simulink model "Save"  (R2020b)
settings: Solver=VariableStepAuto  StartTime=0.0  StopTime=10.0  RelTol=1e-3
values from neighbouring files (symbols this model uses):
  A_2 = [0  0  0; 0  0  0; 0  0  0]    [Angular_gust.mat]    (also in Linear_gust.mat; Real_Values.m = zeros(3); Trial_Script.m = zeros(3); TryingNewAeroCoeffs.m = zeros(3))
  A_AD = [0 0 0 0 0 0 0 0 0 0 0 0 ... (36 elements, 6x6)]    [Angular_gust.mat]    (also in Linear_gust.mat; Real_Values.m = horzcat(A_i, A_ii); Trial_Script.m = horzcat(A_i, A_ii); TryingNewAeroCoeffs.m = horzcat(A_i, A_ii))
  A_kal = [0 0 0 0 0 0 0 0 0 0 0 0 ... (36 elements, 6x6)]    [Angular_gust.mat]    (also in Linear_gust.mat; Real_Values.m = [0 0 0 1 0 0; Trial_Script.m = [0 0 0 1 0 0; TryingNewAeroCoeffs.m = [0 0 0 1 0 0)
  B_2 = [0.0024294842205  2.57653534931e-06  6.44659625064e-05; 0  -0.000916808772026  -2.10833406567e-07; 0  0  -0.000799328564006]    [Angular_gust.mat]    (also in Linear_gust.mat; Real_Values.m = I_inv; Trial_Script.m = I_inv; TryingNewAeroCoeffs.m = I_inv)
  B_AD = [0 0 0 0 0 0 0 0 0 0 0 0 ... (36 elements, 6x6)]    [Angular_gust.mat]    (also in Linear_gust.mat; Real_Values.m = horzcat(B_i, B_ii); Trial_Script.m = horzcat(B_i, B_ii); TryingNewAeroCoeffs.m = horzcat(B_i, B_ii))
  B_kal = [0 0 0 0 0 0 0 0 0 0 0 0 ... (36 elements, 6x6)]    [Angular_gust.mat]    (also in Linear_gust.mat; Real_Values.m = [0 0 0 0 0 0; Trial_Script.m = [0 0 0 0 0 0; TryingNewAeroCoeffs.m = [0 0 0 0 0 0)
  C_2 = [1  0  0; 0  1  0; 0  0  1]    [Angular_gust.mat]    (also in Linear_gust.mat; Real_Values.m = eye(3); Trial_Script.m = eye(3); TryingNewAeroCoeffs.m = eye(3))
  C_AD = [1 0 0 0 0 0 0 1 0 0 0 0 ... (36 elements, 6x6)]    [Angular_gust.mat]    (also in Linear_gust.mat; Real_Values.m = eye(6); Trial_Script.m = eye(6); TryingNewAeroCoeffs.m = eye(6))
  C_D = 0.6    [Angular_gust.mat]    (also in Linear_gust.mat; Real_Values.m; Trial_Script.m; TryingNewAeroCoeffs.m)
  C_kal = [1 0 0 0 0 0 0 1 0 0 0 0 ... (36 elements, 6x6)]    [Angular_gust.mat]    (also in Linear_gust.mat; Real_Values.m = eye(6); Trial_Script.m = eye(6); TryingNewAeroCoeffs.m = eye(6))
  D_2 = [0  0  0; 0  0  0; 0  0  0]    [Angular_gust.mat]    (also in Linear_gust.mat; Real_Values.m = zeros(3); Trial_Script.m = zeros(3); TryingNewAeroCoeffs.m = zeros(3))
  D_AD = [0 0 0 0 0 0 0 0 0 0 0 0 ... (36 elements, 6x6)]    [Angular_gust.mat]    (also in Linear_gust.mat; Real_Values.m = zeros(6); Trial_Script.m = zeros(6); TryingNewAeroCoeffs.m = zeros(6))
  D_kal = [0 0 0 0 0 0 0 0 0 0 0 0 ... (36 elements, 6x6)]    [Angular_gust.mat]    (also in Linear_gust.mat; Real_Values.m = zeros(6); Trial_Script.m = zeros(6); TryingNewAeroCoeffs.m = zeros(6))
  delta_time = 0.0178961433409    [Angular_gust.mat]    (also in Linear_gust.mat; Real_Values.m = time/length(xdata); Trial_Script.m = time/length(xdata); TryingNewAeroCoeffs.m = time/length(xdata))
  Fb1_l = -2600    [Angular_gust.mat]    (also in Linear_gust.mat; Real_Values.m = -260; Trial_Script.m; TryingNewAeroCoeffs.m)
  Fb1_u = 2600    [Angular_gust.mat]    (also in Linear_gust.mat; Real_Values.m = 260; Trial_Script.m; TryingNewAeroCoeffs.m)
  Fb2_l = -2600    [Angular_gust.mat]    (also in Linear_gust.mat; Real_Values.m = -260; Trial_Script.m; TryingNewAeroCoeffs.m)
  Fb2_u = 2600    [Angular_gust.mat]    (also in Linear_gust.mat; Real_Values.m = 260; Trial_Script.m; TryingNewAeroCoeffs.m)
  Fb3_l = -3200    [Angular_gust.mat]    (also in Linear_gust.mat; Real_Values.m = -320; Trial_Script.m; TryingNewAeroCoeffs.m)
  Fb3_u = 3200    [Angular_gust.mat]    (also in Linear_gust.mat; Real_Values.m = 320; Trial_Script.m; TryingNewAeroCoeffs.m)
  Fb4_l = -3200    [Angular_gust.mat]    (also in Linear_gust.mat; Real_Values.m = -320; Trial_Script.m; TryingNewAeroCoeffs.m)
  Fb4_u = 3200    [Angular_gust.mat]    (also in Linear_gust.mat; Real_Values.m = 320; Trial_Script.m; TryingNewAeroCoeffs.m)
  Fc1_l = -300    [Angular_gust.mat]    (also in Linear_gust.mat; Real_Values.m = -100; Trial_Script.m = -3000; TryingNewAeroCoeffs.m)
  Fc1_u = 300    [Angular_gust.mat]    (also in Linear_gust.mat; Real_Values.m = 100; Trial_Script.m = 3000; TryingNewAeroCoeffs.m)
  Fc2_l = -300    [Angular_gust.mat]    (also in Linear_gust.mat; Real_Values.m = -100; Trial_Script.m = -3000; TryingNewAeroCoeffs.m)
  Fc2_u = 300    [Angular_gust.mat]    (also in Linear_gust.mat; Real_Values.m = 100; Trial_Script.m = 3000; TryingNewAeroCoeffs.m)
  Fc3_l = -300    [Angular_gust.mat]    (also in Linear_gust.mat; Real_Values.m = -100; Trial_Script.m = -3000; TryingNewAeroCoeffs.m)
  Fc3_u = 300    [Angular_gust.mat]    (also in Linear_gust.mat; Real_Values.m = 100; Trial_Script.m = 3000; TryingNewAeroCoeffs.m)
  Ft1_l = -5600    [Angular_gust.mat]    (also in Linear_gust.mat; Real_Values.m = -560; Trial_Script.m; TryingNewAeroCoeffs.m)
  Ft1_u = 5600    [Angular_gust.mat]    (also in Linear_gust.mat; Real_Values.m = 560; Trial_Script.m; TryingNewAeroCoeffs.m)
  Ft2_l = -5600    [Angular_gust.mat]    (also in Linear_gust.mat; Real_Values.m = -560; Trial_Script.m; TryingNewAeroCoeffs.m)
  Ft2_u = 5600    [Angular_gust.mat]    (also in Linear_gust.mat; Real_Values.m = 560; Trial_Script.m; TryingNewAeroCoeffs.m)
  Ft3_l = -3200    [Angular_gust.mat]    (also in Linear_gust.mat; Real_Values.m = -320; Trial_Script.m; TryingNewAeroCoeffs.m)
  Ft3_u = 3200    [Angular_gust.mat]    (also in Linear_gust.mat; Real_Values.m = 320; Trial_Script.m; TryingNewAeroCoeffs.m)
  Ft4_l = -3200    [Angular_gust.mat]    (also in Linear_gust.mat; Real_Values.m = -320; Trial_Script.m; TryingNewAeroCoeffs.m)
  Ft4_u = 3200    [Angular_gust.mat]    (also in Linear_gust.mat; Real_Values.m = 320; Trial_Script.m; TryingNewAeroCoeffs.m)
  g = 9.81    [Angular_gust.mat]    (also in Linear_gust.mat; Real_Values.m; Trial_Script.m; TryingNewAeroCoeffs.m)
  m = 941.102    [Angular_gust.mat]    (also in Linear_gust.mat; Real_Values.m; Trial_Script.m = 645; TryingNewAeroCoeffs.m)
  r_0 = [0 0 0]    [Angular_gust.mat]    (also in Linear_gust.mat; Real_Values.m = [0;0;0]; Trial_Script.m = [0;0;0]; TryingNewAeroCoeffs.m = [0;0;0])
  r_cgCatia = [0.0401998 0.00180957 -0.293434]    [Angular_gust.mat]    (also in Linear_gust.mat; Real_Values.m = TcgCatia*r_cgCatia; Trial_Script.m = [2; 0; 0]; TryingNewAeroCoeffs.m = TcgCatia*r_cgCatia)
  rho = 1.225    [Angular_gust.mat]    (also in Linear_gust.mat; Real_Values.m; Trial_Script.m; TryingNewAeroCoeffs.m)
  S = 1.8    [Angular_gust.mat]    (also in Linear_gust.mat; Real_Values.m; Trial_Script.m; TryingNewAeroCoeffs.m)
  t_finalgust = 17.9140394843    [Angular_gust.mat]    (also in Linear_gust.mat; Real_Values.m = time; TryingNewAeroCoeffs.m = time)
  TcgCatia = [1  0  0; 0  -1  0; 0  0  -1]    [Angular_gust.mat]    (also in Linear_gust.mat; Real_Values.m = [1 0 0; Trial_Script.m = [1 0 0; TryingNewAeroCoeffs.m = [1 0 0)
  theta_0 = [0 0 0]    [Angular_gust.mat]    (also in Linear_gust.mat; Real_Values.m = [0;0;0]; Trial_Script.m = [0;0;0]; TryingNewAeroCoeffs.m = [0;0;0])
  time_delay = 0.01    [Angular_gust.mat]    (also in Linear_gust.mat; Real_Values.m = 0.1; Trial_Script.m = 0.1; TryingNewAeroCoeffs.m)
  Tzy_Shard = [6.12323399574e-17  1  1.22464679915e-16; 1  -6.12323399574e-17  -7.49879891331e-33; 0  1.22464679915e-16  -1]    [Angular_gust.mat]    (also in Linear_gust.mat; Real_Values.m = [cos(pi/2) -sin(pi/2) 0; sin(pi/2) cos(pi/2) 0; 0 0 1]*[1 0 ; Trial_Script.m = [cos(pi/2) -sin(pi/2) 0; sin(pi/2) cos(pi/2) 0; 0 0 1]*[1 0 ; TryingNewAeroCoeffs.m = [cos(pi/2) -sin(pi/2) 0; sin(pi/2) cos(pi/2) 0; 0 0 1]*[1 0 )
  u0_final = 23.9559    [Angular_gust.mat]    (also in Linear_gust.mat; Real_Values.m = u_0(length(u_0)); TryingNewAeroCoeffs.m = u_0(length(u_0)))
  u1_final = -0.480858    [Angular_gust.mat]    (also in Linear_gust.mat; Real_Values.m = u_1(length(u_1)); TryingNewAeroCoeffs.m = u_1(length(u_1)))
  u2_final = -0.725589    [Angular_gust.mat]    (also in Linear_gust.mat; Real_Values.m = u_2(length(u_2)); TryingNewAeroCoeffs.m = u_2(length(u_2)))
  u_0 = [24.7775 24.7775 24.7775 24.7775 24.7775 24.7775 24.7775 24.7775 24.7775 24.7775 24.7775 24.7775 ... (1001 elements, 1001x1)]    [Angular_gust.mat]    (also in Linear_gust.mat; Real_Values.m = a(1:d_shard,1); Trial_Script.m = a(1:d_shard,1); TryingNewAeroCoeffs.m = a(1:d_shard,1))
  u_1 = [0.712897 0.712897 0.712897 0.712897 0.712897 0.712897 0.712897 0.712897 0.712897 0.712897 0.712897 0.712897 ... (1001 elements, 1001x1)]    [Angular_gust.mat]    (also in Linear_gust.mat; Real_Values.m = a(1:d_shard,2); Trial_Script.m = a(1:d_shard,2); TryingNewAeroCoeffs.m = a(1:d_shard,2))
  u_2 = [-0.504815 -0.504815 -0.504815 -0.504815 -0.504815 -0.504815 -0.504815 -0.504815 -0.504815 -0.504815 -0.504815 -0.504815 ... (1001 elements, 1001x1)]    [Angular_gust.mat]    (also in Linear_gust.mat; Real_Values.m = a(1:d_shard,3); Trial_Script.m = a(1:d_shard,3); TryingNewAeroCoeffs.m = a(1:d_shard,3))
  v_0 = [0 0 0]    [Angular_gust.mat]    (also in Linear_gust.mat; Real_Values.m = [0;0;0]; Trial_Script.m = [0;0;0]; TryingNewAeroCoeffs.m = [0;0;0])
  ZI_Cx = [4.10002314469 4.10486511138 4.10970707807 4.11454904475 4.11939101144 4.12423297813 4.12907494481 4.1339169115 4.13875887819 4.14360084487 4.14844281156 4.15328477825 ... (65341 elements, 361x181)]    [Angular_gust.mat]    (also in Linear_gust.mat; Real_Values.m = model_Cx(XI_Cx, YI_Cx); Trial_Script.m = model_Cx(XI_Cx, YI_Cx); TryingNewAeroCoeffs.m = model_Cx(XI_Cx, YI_Cx))
  ZI_Cy = [5.10662222372 5.15407485934 5.20152749496 5.24898013059 5.29643276621 5.34388540184 5.39133803746 5.43879067308 5.48624330871 5.53369594433 5.58114857996 5.62860121558 ... (65341 elements, 361x181)]    [Angular_gust.mat]    (also in Linear_gust.mat; Real_Values.m = model_Cy(XI_Cy, YI_Cy); Trial_Script.m = model_Cy(XI_Cy, YI_Cy); TryingNewAeroCoeffs.m = model_Cy(XI_Cy, YI_Cy))
  ZI_Cz = [-10.5947720774 -10.6317912004 -10.6688103235 -10.7058294465 -10.7428485695 -10.7798676926 -10.8168868156 -10.8539059387 -10.8909250617 -10.9279441847 -10.9649633078 -11.0019824308 ... (65341 elements, 361x181)]    [Angular_gust.mat]    (also in Linear_gust.mat; Real_Values.m = model_Cz(XI_Cz, YI_Cz); Trial_Script.m = model_Cz(XI_Cz, YI_Cz); TryingNewAeroCoeffs.m = model_Cz(XI_Cz, YI_Cz))
  ZI_p = [6.05111971338 6.06712776392 6.08313581446 6.099143865 6.11515191553 6.13115996607 6.14716801661 6.16317606715 6.17918411769 6.19519216823 6.21120021877 6.22720826931 ... (65341 elements, 361x181)]    [Angular_gust.mat]    (also in Linear_gust.mat; Real_Values.m = model_p(XI_p, YI_p); Trial_Script.m = model_p(XI_p, YI_p); TryingNewAeroCoeffs.m = model_p(XI_p, YI_p))
  ZI_q = [0.071083987219 0.054175962948 0.0372679386771 0.0203599144061 0.00345189013513 -0.0134561341358 -0.0303641584068 -0.0472721826778 -0.0641802069487 -0.0810882312197 -0.0979962554907 -0.114904279762 ... (65341 elements, 361x181)]    [Angular_gust.mat]    (also in Linear_gust.mat; Real_Values.m = model_q(XI_q, YI_q); Trial_Script.m = model_q(XI_q, YI_q); TryingNewAeroCoeffs.m = model_q(XI_q, YI_q))
  ZI_r = [-1.8762921931 -1.88364224017 -1.89099228723 -1.8983423343 -1.90569238136 -1.91304242842 -1.92039247549 -1.92774252255 -1.93509256961 -1.94244261668 -1.94979266374 -1.95714271081 ... (65341 elements, 361x181)]    [Angular_gust.mat]    (also in Linear_gust.mat; Real_Values.m = model_r(XI_r, YI_r); Trial_Script.m = model_r(XI_r, YI_r); TryingNewAeroCoeffs.m = model_r(XI_r, YI_r))
undefined symbols (not defined in the file or in its folder): Continuous, Time
libraries: dspsigops x11, simulink x7, pid_lib x3, fuzblock x3, dspindex x3, ctrlSharedLib x2, sharedutil x1, mpclib x1, dspmathops x1, cstblocks x1
(part 2 of 2)

== system Save/Propulsion commands module/Subsystem4 ==
  In1 : Inport
  Fy_actual : Inport  Port=2
  Fz_actual : Inport  Port=3
  In4 : Inport  Port=4
  In5 : Inport  Port=5
  In6 : Inport  Port=6
  T_Vd : Inport  Port=7
  Constant : Constant  Value=[0;1;1]
  Matrix Multiply : Product  Multiplication=Matrix(*)
  Mux : Mux  Inputs=3
  Mux1 : Mux  Inputs=3
  Product : Product
  Scope : Scope
  F_c : Outport
  y : Outport  Port=2
  wires:
  In1/1 -> Mux/1
  Fy_actual/1 -> Mux/2
  Fz_actual/1 -> Mux/3
  Product/1 -> Scope/1, F_c/1  "Fc(t-tau)_actual"
  Mux/1 -> Matrix Multiply/2
  Mux1/1 -> y/1  "Mc(t-tau)_actual"
  In4/1 -> Mux1/1  "M_x_acc"
  In5/1 -> Mux1/2  "M_y_acc"
  In6/1 -> Mux1/3  "M_z_acc"
  T_Vd/1 -> Matrix Multiply/1
  Constant/1 -> Product/1
  Matrix Multiply/1 -> Product/2  "Fc(t-tau)_actual"

== system Save/Propulsion commands module/Top and Bottom including weight counteraction ==
  F_b : Inport
  In2 : Inport  Port=2
  Add : Sum
  Add1 : Sum
  Constant : Constant  Value=m*g
  Gain : Gain  Gain=1/8
  Mux : Mux
  Scope : Scope
  To Workspace : ToWorkspace  VariableName=Ft_inclift  SaveFormat=Timeseries  SampleTime=-1
  To Workspace1 : ToWorkspace  VariableName=Fb_inclift  SaveFormat=Timeseries  SampleTime=-1
  wires:
  Constant/1 -> Mux/4, Mux/3, Mux/2, Mux/1
  Add1/1 -> To Workspace1/1
  F_b/1 -> Add1/1  "F_b"
  In2/1 -> Add/1  "F_t"
  Add/1 -> Scope/1, To Workspace/1
  Gain/1 -> Add1/2, Add/2
  Mux/1 -> Gain/1

== system Save/Subsystem/Drag1 ==
  note: Change to C_D and S per side
  In1 : Inport
  Constant1 : Constant  Value=2
  Constant4 : Constant  Value=0.5*rho*C_D*S
  Demux : Demux  Outputs=3
  Gain : Gain  Gain=0
  Mux : Mux  Inputs=3
  Power : Math  Operator=pow  SaturateOnIntegerOverflow=on
  Power1 : Math  Operator=pow  SaturateOnIntegerOverflow=on
  Power2 : Math  Operator=pow  SaturateOnIntegerOverflow=on
  Product1 : Product
  Out1 : Outport
  drag : Outport  Port=2
  wires:
  Constant1/1 -> Power2/2, Power1/2, Power/2
  Power2/1 -> Mux/3
  Power/1 -> Gain/1
  In1/1 -> Demux/1
  Demux/1 -> Power/1
  Demux/3 -> Power2/1
  Demux/2 -> Power1/1
  Power1/1 -> Mux/2
  Constant4/1 -> Product1/2
  Mux/1 -> Out1/1, Product1/1
  Product1/1 -> drag/1  "drag"
  Gain/1 -> Mux/1

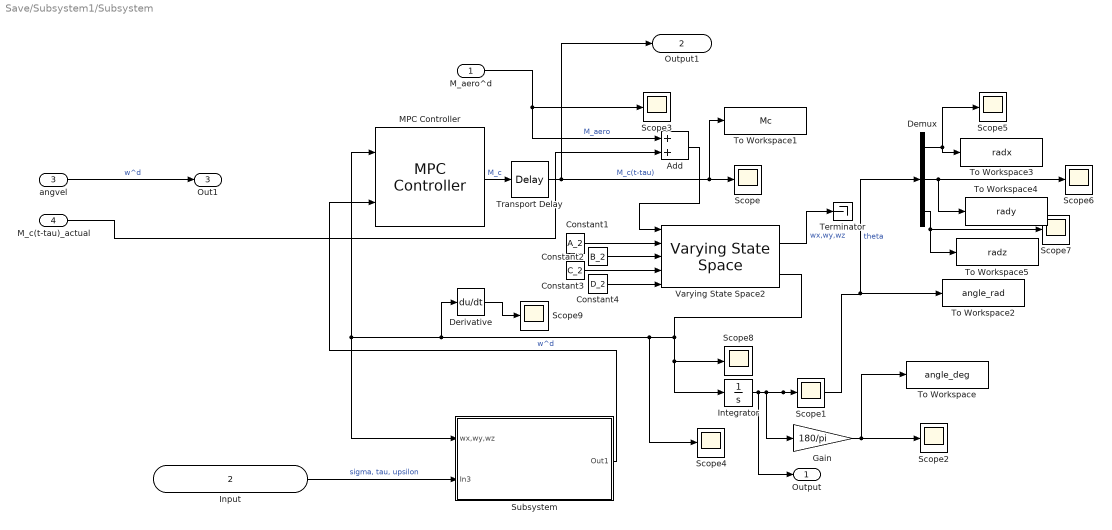
== system Save/Subsystem1/Subsystem ==
  M_aero^d : Inport
  Input : Inport  Port=2
  angvel : Inport  Port=3
  M_c(t-tau)_actual : Inport  Port=4
  Add : Sum
  Constant1 : Constant  Value=A_2
  Constant2 : Constant  Value=B_2
  Constant3 : Constant  Value=C_2
  Constant4 : Constant  Value=D_2
  Demux : Demux  Outputs=3
  Derivative : Derivative
  Gain : Gain  Gain=180/pi
  Integrator : Integrator  InitialCondition=[0;0;0]
  MPC Controller : mpclib/MPC Controller  SCDEnableBlockLinearizationSpecification=on  mpcobj=MPCDesignerSession.AppData.Controllers.MPC  is_multiple=0  enable_value=0  return_u0=off  updateMPCinCallerWorkspace=on  md_inport=off  mv_inport=off  uref_inport=off  return_cost=off  return_mvseq=off  return_qpstatus=off  return_xseq=off  return_state=off  return_ovseq=off  state_inport=off  umin_inport=off  umax_inport=off  ymin_inport=off  ymax_inport=off  cc_inport=off  ywt_inport=off  uwt_inport=off  duwt_inport=off  rhoeps_inport=off  pm_inport=off  MaximumP=10  HorizonChoice=FixedHorizon  n_ts=0.1  n_p=10  n_mv=3  n_md=0  n_ud=0  n_mo=3  n_uo=0  BlockDataType=double  SampleTimeInherited=off  switch_inport=off
  Scope{,1..9} (10 alike) : Scope
  Subsystem : Subsystem
  Terminator : Terminator
  To Workspace : ToWorkspace  VariableName=angle_deg  SaveFormat=Timeseries  SampleTime=-1
  To Workspace1 : ToWorkspace  VariableName=Mc  SaveFormat=Timeseries  SampleTime=-1
      settings: Save2DSignal=2-D array (concatenate along first dimension)
  To Workspace2 : ToWorkspace  VariableName=angle_rad  SaveFormat=Timeseries  SampleTime=-1
  To Workspace3 : ToWorkspace  VariableName=radx  SaveFormat=Timeseries  SampleTime=-1
  To Workspace4 : ToWorkspace  VariableName=rady  SaveFormat=Timeseries  SampleTime=-1
  To Workspace5 : ToWorkspace  VariableName=radz  SaveFormat=Timeseries  SampleTime=-1
  Transport Delay : TransportDelay  DelayTime=0.1
  Varying State Space2 : cstblocks/Linear Parameter Varying/Varying State Space  x0=0  xNames=''  OutputX=on  OutputDX=off
  Output : Outport
  Output1 : Outport  Port=2
  Out1 : Outport  Port=3
  wires:
  Demux/3 -> To Workspace5/1, Scope7/1
  Subsystem/1(Out1) -> MPC Controller/2
  Constant1/1 -> Varying State Space2/2
  MPC Controller/1 -> Transport Delay/1  "M_c"
  Derivative/1 -> Scope9/1
  Demux/1 -> Scope5/1, To Workspace3/1
  Constant4/1 -> Varying State Space2/5
  Demux/2 -> To Workspace4/1, Scope6/1
  Gain/1 -> To Workspace/1, Scope2/1
  Integrator/1 -> Demux/1, To Workspace2/1, Scope1/1, Gain/1, Output/1  "theta"
  Input/1 -> Subsystem/2(In3)  "sigma, tau, upsilon"
  Add/1 -> Varying State Space2/1
  Varying State Space2/1 -> Terminator/1  "wx,wy,wz"
  Constant2/1 -> Varying State Space2/3
  Constant3/1 -> Varying State Space2/4
  Transport Delay/1 -> Output1/1, To Workspace1/1, Scope/1  "M_c(t-tau)"
  M_aero^d/1 -> Scope3/1, Add/1  "M_aero"
  Varying State Space2/2 -> Scope8/1, Integrator/1, MPC Controller/1, Subsystem/1(wx,wy,wz), Derivative/1, Scope4/1  "w^d"
  angvel/1 -> Out1/1  "w^d"
  M_c(t-tau)_actual/1 -> Add/2

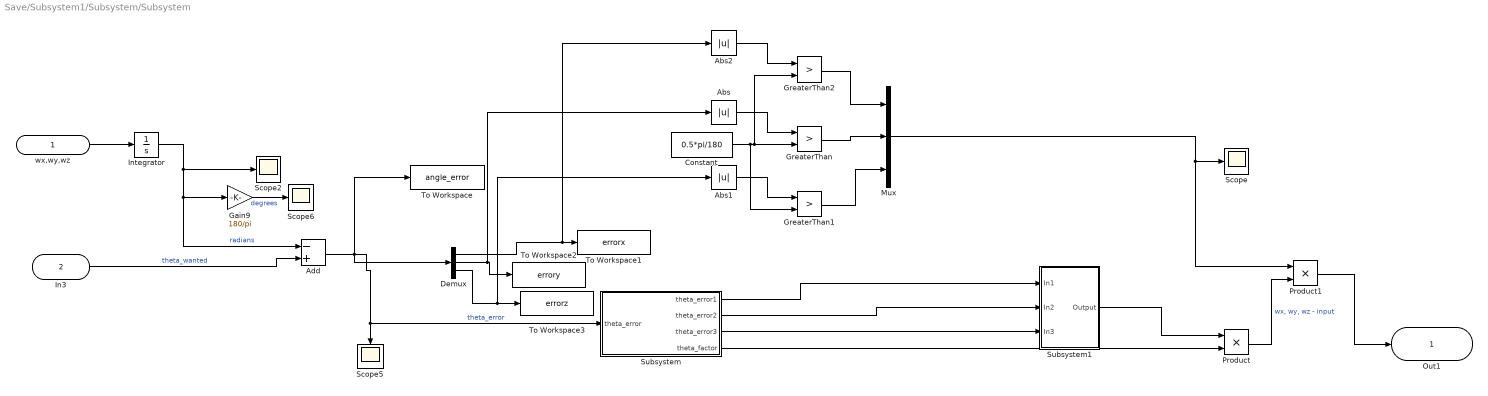
== system Save/Subsystem1/Subsystem/Subsystem ==
  wx,wy,wz : Inport
  In3 : Inport  Port=2
  Abs : Abs
  Abs1 : Abs
  Abs2 : Abs
  Add : Sum  Inputs=-+
  Constant : Constant  Value=0.5*pi/180
  Demux : Demux  Outputs=3
  Gain9 : Gain  Gain=180/pi
  GreaterThan : RelationalOperator  Operator=>  OutDataTypeStr=boolean  RndMeth=Simplest
  GreaterThan1 : RelationalOperator  Operator=>  OutDataTypeStr=boolean  RndMeth=Simplest
  GreaterThan2 : RelationalOperator  Operator=>  OutDataTypeStr=boolean  RndMeth=Simplest
  Integrator : Integrator  InitialCondition=theta_0
  Mux : Mux  Inputs=3
  Product : Product
  Product1 : Product
  Scope{,2,5..6} (4 alike) : Scope
  Subsystem : Subsystem
  Subsystem1 : Subsystem
  To Workspace : ToWorkspace  VariableName=angle_error  SampleTime=-1
  To Workspace1 : ToWorkspace  VariableName=errorx  SaveFormat=Timeseries  SampleTime=-1
      settings: Save2DSignal=2-D array (concatenate along first dimension)
  To Workspace2 : ToWorkspace  VariableName=errory  SaveFormat=Timeseries  SampleTime=-1
  To Workspace3 : ToWorkspace  VariableName=errorz  SaveFormat=Timeseries  SampleTime=-1
  Out1 : Outport
  wires:
  Integrator/1 -> Add/1, Gain9/1, Scope2/1  "radians"
  Add/1 -> To Workspace/1, Demux/1, Subsystem/1(theta_error), Scope5/1  "theta_error"
  Gain9/1 -> Scope6/1  "degrees"
  In3/1 -> Add/2  "theta_wanted"
  Product/1 -> Product1/2  "wx, wy, wz - input"
  wx,wy,wz/1 -> Integrator/1
  Subsystem/4(theta_factor) -> Product/2
  Demux/2 -> Abs/1, To Workspace2/1
  Demux/3 -> Abs1/1, To Workspace3/1
  Demux/1 -> Abs2/1, To Workspace1/1
  Subsystem/1(theta_error1) -> Subsystem1/1(In1)
  Subsystem/2(theta_error2) -> Subsystem1/2(In2)
  Subsystem/3(theta_error3) -> Subsystem1/3(In3)
  Subsystem1/1(Output) -> Product/1
  Abs/1 -> GreaterThan/1
  Constant/1 -> GreaterThan1/2, GreaterThan2/2, GreaterThan/2
  Abs1/1 -> GreaterThan1/1
  Abs2/1 -> GreaterThan2/1
  GreaterThan2/1 -> Mux/1
  GreaterThan/1 -> Mux/2
  GreaterThan1/1 -> Mux/3
  Mux/1 -> Scope/1, Product1/1
  Product1/1 -> Out1/1

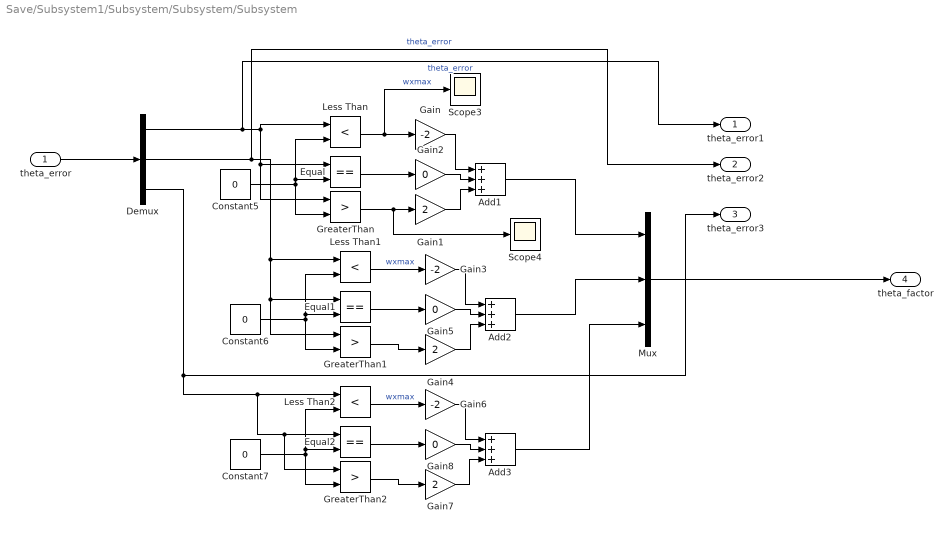
== system Save/Subsystem1/Subsystem/Subsystem/Subsystem ==
  theta_error : Inport
  Add1 : Sum  Inputs=+++
  Add2 : Sum  Inputs=+++
  Add3 : Sum  Inputs=+++
  Constant5 : Constant  Value=0
  Constant6 : Constant  Value=0
  Constant7 : Constant  Value=0
  Demux : Demux  Outputs=3
  Equal : RelationalOperator  Operator===  OutDataTypeStr=boolean  RndMeth=Simplest
  Equal1 : RelationalOperator  Operator===  OutDataTypeStr=boolean  RndMeth=Simplest
  Equal2 : RelationalOperator  Operator===  OutDataTypeStr=boolean  RndMeth=Simplest
  Gain : Gain  Gain=-2
  Gain1 : Gain  Gain=2
  Gain2 : Gain  Gain=0
  Gain3 : Gain  Gain=-2
  Gain4 : Gain  Gain=2
  Gain5 : Gain  Gain=0
  Gain6 : Gain  Gain=-2
  Gain7 : Gain  Gain=2
  Gain8 : Gain  Gain=0
  GreaterThan : RelationalOperator  Operator=>  OutDataTypeStr=boolean  RndMeth=Simplest
  GreaterThan1 : RelationalOperator  Operator=>  OutDataTypeStr=boolean  RndMeth=Simplest
  GreaterThan2 : RelationalOperator  Operator=>  OutDataTypeStr=boolean  RndMeth=Simplest
  Less Than : RelationalOperator  Operator=<  OutDataTypeStr=boolean  RndMeth=Simplest
  Less Than1 : RelationalOperator  Operator=<  OutDataTypeStr=boolean  RndMeth=Simplest
  Less Than2 : RelationalOperator  Operator=<  OutDataTypeStr=boolean  RndMeth=Simplest
  Mux : Mux  Inputs=3
  Scope3 : Scope
  Scope4 : Scope
  theta_error1 : Outport
  theta_error2 : Outport  Port=2
  theta_error3 : Outport  Port=3
  theta_factor : Outport  Port=4
  wires:
  Add1/1 -> Mux/1
  Constant5/1 -> Equal/2, Less Than/2, GreaterThan/2
  Equal2/1 -> Gain8/1
  Demux/1 -> theta_error1/1, GreaterThan/1, Equal/1, Less Than/1  "theta_error"
  GreaterThan2/1 -> Gain7/1
  Gain1/1 -> Add1/3
  Gain7/1 -> Add3/3
  Less Than1/1 -> Gain3/1  "wxmax"
  Gain6/1 -> Add3/1
  Equal/1 -> Gain2/1
  Gain5/1 -> Add2/2
  Add3/1 -> Mux/3
  GreaterThan/1 -> Scope4/1, Gain1/1
  Constant6/1 -> Equal1/2, Less Than1/2, GreaterThan1/2
  Demux/3 -> theta_error3/1, GreaterThan2/1, Equal2/1, Less Than2/1
  Gain3/1 -> Add2/1
  Constant7/1 -> Equal2/2, Less Than2/2, GreaterThan2/2
  Equal1/1 -> Gain5/1
  Gain8/1 -> Add3/2
  Gain4/1 -> Add2/3
  GreaterThan1/1 -> Gain4/1
  Gain/1 -> Add1/1
  Demux/2 -> theta_error2/1, GreaterThan1/1, Equal1/1, Less Than1/1  "theta_error"
  Gain2/1 -> Add1/2
  Add2/1 -> Mux/2
  Less Than/1 -> Scope3/1, Gain/1  "wxmax"
  Less Than2/1 -> Gain6/1  "wxmax"
  theta_error/1 -> Demux/1
  Mux/1 -> theta_factor/1

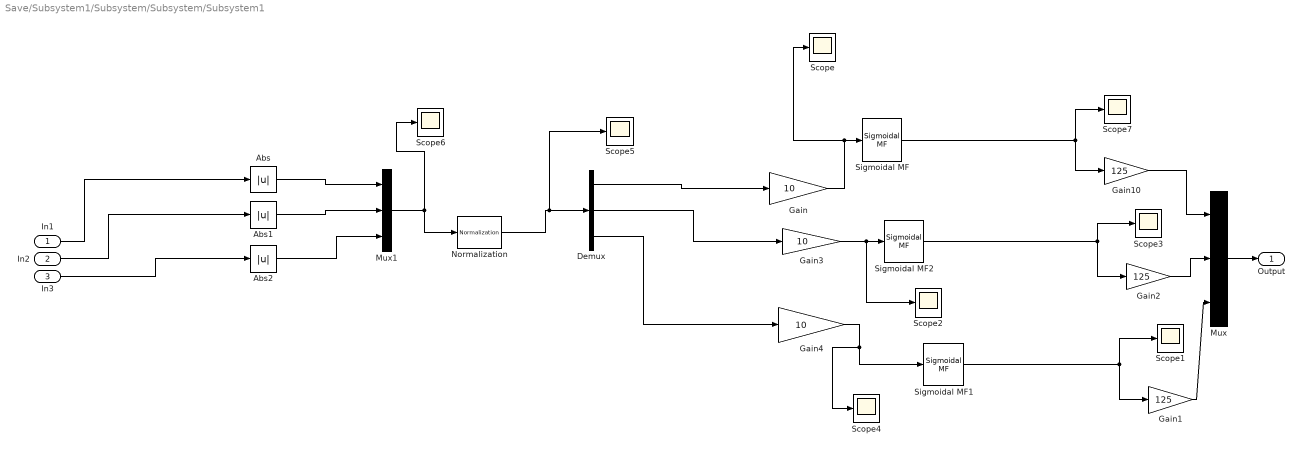
== system Save/Subsystem1/Subsystem/Subsystem/Subsystem1 ==
  In1 : Inport
  In2 : Inport  Port=2
  In3 : Inport  Port=3
  Abs : Abs
  Abs1 : Abs
  Abs2 : Abs
  Demux : Demux  Outputs=3
  Gain : Gain  Gain=10
  Gain1 : Gain  Gain=125
  Gain10 : Gain  Gain=125
  Gain2 : Gain  Gain=125
  Gain3 : Gain  Gain=10
  Gain4 : Gain  Gain=10
  Mux : Mux  Inputs=3
  Mux1 : Mux  Inputs=3
  Normalization : dspmathops/Normalization  NormType=Squared 2-norm  Bias=1e-10  NormOver=Each column  Dimension=1  roundingMode=Floor  overflowMode=off  accumDataTypeStr=Inherit: Same as product output  accumLastDataTypeStr=Inherit: Same as product output  outputDataTypeStr=Inherit: Same as product output  outputMin=[]  outputMax=[]  outputLastDataTypeStr=Inherit: Same as product output
  Scope{,1..7} (8 alike) : Scope
  Sigmoidal MF : fuzblock/Membership  Functions/Sigmoidal MF  a=10^(-8)  c=1000
      settings: SourceProductBaseCode=FL
  Sigmoidal MF1 : fuzblock/Membership  Functions/Sigmoidal MF  a=10^(-8)  c=1000
      settings: SourceProductBaseCode=FL
  Sigmoidal MF2 : fuzblock/Membership  Functions/Sigmoidal MF  a=10^(-8)  c=1000
      settings: SourceProductBaseCode=FL
  Output : Outport
  wires:
  Gain2/1 -> Mux/2
  Gain10/1 -> Mux/1
  Sigmoidal MF1/1 -> Gain1/1, Scope1/1
  Sigmoidal MF/1 -> Gain10/1, Scope7/1
  Sigmoidal MF2/1 -> Gain2/1, Scope3/1
  Gain/1 -> Scope/1, Sigmoidal MF/1
  Gain1/1 -> Mux/3
  Gain3/1 -> Scope2/1, Sigmoidal MF2/1
  In2/1 -> Abs1/1
  In1/1 -> Abs/1
  In3/1 -> Abs2/1
  Mux/1 -> Output/1
  Abs/1 -> Mux1/1
  Abs1/1 -> Mux1/2
  Gain4/1 -> Scope4/1, Sigmoidal MF1/1
  Abs2/1 -> Mux1/3
  Demux/3 -> Gain4/1
  Demux/1 -> Gain/1
  Demux/2 -> Gain3/1
  Mux1/1 -> Normalization/1, Scope6/1
  Normalization/1 -> Scope5/1, Demux/1

== matlab function Save/Transformation Subsystem/MATLAB Function2 ==
  data: theta_x input; Transformation_Mat output; theta_y input; theta_z input
function Transformation_Mat  = Euler(theta_x, theta_y, theta_z)

a = cos(theta_x)*cos(theta_z);
b = cos(theta_x)*sin(theta_z);
c = - sin(theta_x);
d = sin(theta_y)*sin(theta_x)*cos(theta_z) - cos(theta_y)*sin(theta_z);
e = sin(theta_y)*sin(theta_x)*sin(theta_z) + cos(theta_y)*cos(theta_z);
f = sin(theta_y)*cos(theta_x);
g = cos(theta_y)*sin(theta_x)*cos(theta_z) + sin(theta_y)*sin(theta_z);
h = cos(theta_y)*sin(theta_x)*sin(theta_z) - sin(theta_y)*cos(theta_z);
i = cos(theta_y)*cos(theta_x);

Transformation_Mat = [a b c;
    d e f;
    g h i];


end

== matlab function Save/GPS model/GPS Model ==
  settings: updateMethod=DISCRETE
  data: position input; newposition output
function newposition  = gps(position)

    % Input: position
    % Output: position with gps accuracies inclduded
    mu = 0; 
    sigma = 0.015;

    r1 = normrnd(mu, sigma);
    r2 = normrnd(mu, sigma);
    r3 = normrnd(mu, sigma);

    newposition = [0,0,0];

    newposition(1) = position(1) + r1;
    newposition(2) = position(2) + r2;
    newposition(3) = position(3) + r3;

end

== matlab function Save/Transformation Subsystem/MATLAB Function1 ==
  data: theta_x input; Transformation_Mat output; theta_y input; theta_z input
function Transformation_Mat  = Euler(theta_x, theta_y, theta_z)

a = cos(theta_x)*cos(theta_z);
b = cos(theta_x)*sin(theta_z);
c = - sin(theta_x);
d = sin(theta_y)*sin(theta_x)*cos(theta_z) - cos(theta_y)*sin(theta_z);
e = sin(theta_y)*sin(theta_x)*sin(theta_z) + cos(theta_y)*cos(theta_z);
f = sin(theta_y)*cos(theta_x);
g = cos(theta_y)*sin(theta_x)*cos(theta_z) + sin(theta_y)*sin(theta_z);
h = cos(theta_y)*sin(theta_x)*sin(theta_z) - sin(theta_y)*cos(theta_z);
i = cos(theta_y)*cos(theta_x);

Transformation_Mat = [a b c;
    d e f;
    g h i];


end

== matlab function Save/Propulsion commands module/Propeller firing function/MATLAB Function ==
  data: F_wanted input; F_c output; M_wanted input; F_t output; F_b output
function [F_c, F_t, F_b] = propeller_required_forces_control(F_wanted, M_wanted)

%% Load propeller arms data
xc_1 = 0.1;
yc_1 = 0;
zc_1 = 0.3;
xc_2 = 0.1;
yc_2 = 0;
zc_2 = 0.32;
xc_3 = 0.11;
yc_3 = 0;
zc_3 = 0.31;

xt_1 = 0.2;
yt_1 = 0.2;
zt_1 = 1;
xt_2 = 0.2;
yt_2 = 0.2;
zt_2 = 1;
xt_3 = 0.2;
yt_3 = 0.2;
zt_3 = 1;
xt_4 = 0.2;
yt_4 = 0.2;
zt_4 = 1;

xb_1 = 0.4;
yb_1 = 0.3;
zb_1 = 1.2;
xb_2 = 0.4;
yb_2 = 0.3;
zb_2 = 1.2;
xb_3 = 0.4;
yb_3 = 0.3;
zb_3 = 1.2;
xb_4 = 0.4;
yb_4 = 0.3;
zb_4 = 1.2;

%% Decompose force and moment input

F_x = F_wanted(1);
F_y = F_wanted(2);

F_z = F_wanted(3);

M_x = M_wanted(1);
M_y = M_wanted(2);
M_z = M_wanted(3);

%% Find control forces
A_control = [1 1 1;
    zc_1 -zc_2 -zc_3;
    -xc_1 -xc_2 xc_3];
A_cinv = inv(A_control);
force_control = [F_y; M_x; M_z];
controlvec = A_cinv*force_control;
F_c1 = controlvec(1);
F_c2 = controlvec(2);
F_c3 = controlvec(3);

%% Find top and bottom forces
A_tb = [-1 -1;
    2*(xt_1 + xb_1) -2*(xt_3 + xb_3)];
A_tbinv = inv(A_tb);
force_tb = [F_z; M_y];
tbvec = A_tbinv * force_tb;
f_front = tbvec(1);
F_t1 = f_front/4;
F_t2 = f_front/4;
F_b1 = f_front/4;
F_b2 = f_front/4;
f_back = tbvec(2);
F_t3 = f_back/4;
F_t4 = f_back/4;
F_b3 = f_back/4;
F_b4 = f_back/4;



%% Make matrix
F_c = [F_c1; F_c2; F_c3];
F_t = [F_t1; F_t2; F_t3; F_t4];
F_b = [F_b1; F_b2; F_b3; F_b4];
end

== matlab function Save/Subsystem2/MATLAB Function ==
  settings: updateMethod=DISCRETE
  data: angvel input; accelData output; acc input
function accelData = accelerometer(angvel, acc)

    %
    % Create gyroscope sensor object
    params = accelparams;
    
    % Parameters for simulated signal
    N = 1;       % Number of samples
    Fs = 100000;       % Sampling rate
    %Fc = 0.25;      % Sinusoidal frequency
    
    
    % Create arrays
    t = (0:(1/Fs):((N-1)/Fs)).';
    acc = acc;          %Input accelerations
    orient = quaternion.ones(N, 1);
    angvel = angvel;
    
    % Generate acceleration data
    imu = imuSensor('SampleRate', Fs, 'Accelerometer', params);
    imu.Accelerometer.MeasurementRange = 1000;   % Maximum acceleration accelerometer can measure
    imu.Accelerometer.Resolution = 1/Fs;           % Step size of digital measurements
    
    % Biases
    imu.Accelerometer.BiasInstability = 0.000000000001; 7.5 / 1000 * 9.81;
    imu.Accelerometer.NoiseDensity = 0.000000000001;%150 / 1000 / 1000 * 9.81 /10; 
    imu.Accelerometer.TemperatureBias = 50 / 1000 / 1000 * 9.81;
    
  
    
    accelData = imu(acc, angvel, orient);
    
    accelData(:,3) = accelData(:,3) - 9.81;

    accelData(:,1) = accelData(:,1) * -1;
    accelData(:,2) = accelData(:,2) * -1;
    accelData(:,3) = accelData(:,3) * -1;

end

== matlab function Save/Gyroscope Model/MATLAB Function ==
  settings: updateMethod=DISCRETE
  data: xvel input; yvel input; zvel input; gyroData output; acc input
function gyroData  = fungyroscope(xvel, yvel, zvel, acc)
   
    % Create gyroscope sensor object
    params = gyroparams;         
    
    % Parameters for simulated signal
    N = 1;       % Number of samples
    Fs = 100;       % Sampling rate
    Fc = 0.25;      % Sinusoidal frequency
    
    % Create arrays
    t = (0:(1/Fs):((N-1)/Fs)).';
    acc = acc;          % Input accelerations
    angvel = [xvel,yvel,zvel];
    %angvel(:,1) = 8*sin(2*pi*Fc*t);
    
    % Generate gyroscopic data
    imu = imuSensor('SampleRate', Fs, 'Gyroscope', params);
    imu.Gyroscope.MeasurementRange = 6.5;   % Maximum angular velocity gyroscope can measure
    imu.Gyroscope.Resolution = 1/Fs;           % Step size of digital measurements
    
    % Biases
    
    imu.Gyroscope.BiasInstability = 0.12 * 3.14159 / 180;       % rad/hr
    imu.Gyroscope.NoiseDensity = 0.15 * 3.14159 / 180;          % rad/s
    imu.Gyroscope.RandomWalk = 0.017 * 3.14159 / 180;           % rad/sqrt(hr)
    imu.Gyroscope.TemperatureBias = 0.25 * 3.14159 / 180;       % rad/s
    %imu.Gyroscope.AccelerationBias = 0.3;
    
    % Define real accelerations
    %acc(:,1) = 1;
    [~, gyroData] = imu(acc, angvel, eye(3));
    

end

== matlab function Save/Propulsion commands module/Subsystem3/MATLAB Function ==
  data: Fc input; Fx_acc output; Ft input; Fb input; Fy_acc output; Fz_acc output; Mx_acc output; My_acc output; Mz_acc output
function [Fx_acc,Fy_acc, Fz_acc, Mx_acc, My_acc, Mz_acc] = fcn(Fc, Ft, Fb)

%% Load propeller arms data
xc_1 = 0.1;
yc_1 = 0;
zc_1 = 0.3;
xc_2 = 0.1;
yc_2 = 0;
zc_2 = 0.32;
xc_3 = 0.11;
yc_3 = 0;
zc_3 = 0.31;

xt_1 = 0.2;
yt_1 = 0.2;
zt_1 = 1;
xt_2 = 0.2;
yt_2 = 0.2;
zt_2 = 1;
xt_3 = 0.2;
yt_3 = 0.2;
zt_3 = 1;
xt_4 = 0.2;
yt_4 = 0.2;
zt_4 = 1;

xb_1 = 0.4;
yb_1 = 0.3;
zb_1 = 1.2;
xb_2 = 0.4;
yb_2 = 0.3;
zb_2 = 1.2;
xb_3 = 0.4;
yb_3 = 0.3;
zb_3 = 1.2;
xb_4 = 0.4;
yb_4 = 0.3;
zb_4 = 1.2;


%% Split vectors
Fx_acc = 0;

A_control = [1 1 1;
    zc_1 -zc_2 -zc_3;
    -xc_1 -xc_2 xc_3];
ab_control = A_control*Fc;
Fy_acc = ab_control(1);
Mx_acc = ab_control(2);
Mz_acc = ab_control(3);

A_tb = [-1 -1;
    2*(xt_1 + xb_1) -2*(xt_3 + xb_3)];
F_front = Ft(1) + Ft(2) + Fb(1) + Fb(2);
F_back = Ft(3) + Ft(4) + Fb(3) + Fb(4);
Ftb_vec = [F_front; F_back];
Ab_tb = A_tb*Ftb_vec;

Fz_acc = Ab_tb(1);
My_acc = Ab_tb(2);

end

== matlab function Save/Shard Case/MATLAB Function ==
  data: t input; u_0 output; u0 input; u1 input; u2 input; deltat input; u_1 output; u_2 output
function [u_0, u_1, u_2] = fcn(t, u0, u1, u2, deltat)

point = (t+deltat)/deltat;
point = round(point);
if point > length(u0)
    u_0 = u0(length(u0));
    u_1 = u1(length(u1));
    u_2 = u2(length(u2));
else
    u_0 = u0(point);
    u_1 = u1(point);
    u_2 = u2(point);
end

end
